simulink model "StateFlow_Control"  (R2025b)
settings: Solver=VariableStepAuto  StartTime=0.0  StopTime=514*8  RelTol=1e-3
libraries: slpidlib x1, simulink x1
settings Model: Creator=acer  LastModifiedBy=acer

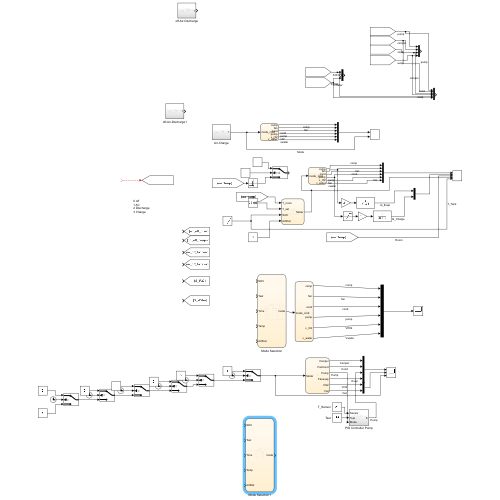
[thumbnail: Simulink's stored preview of the top-level diagram]
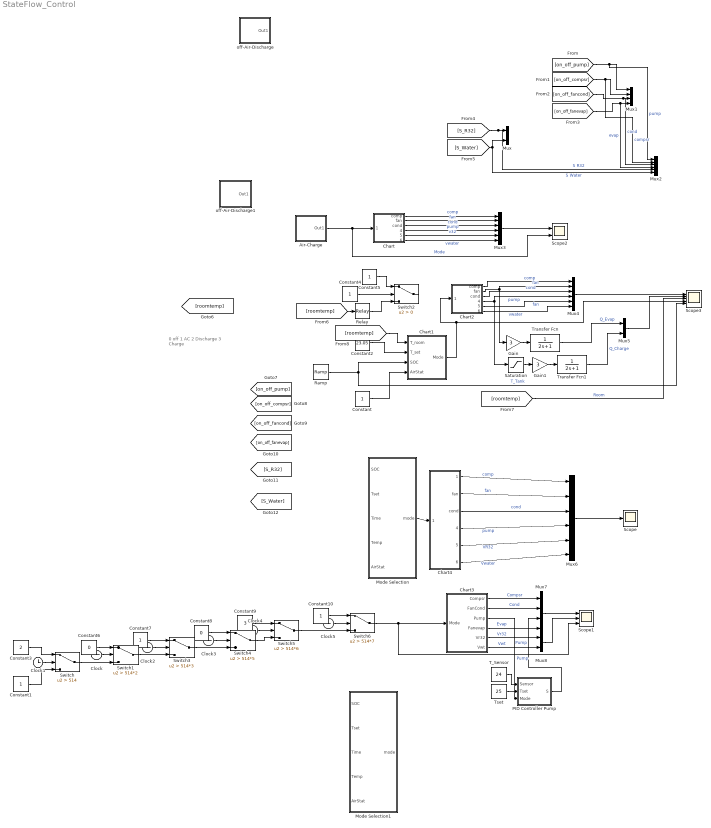
== system StateFlow_Control ==
  note: 0 off
      | 1 AC
      | 2 Discharge
      | 3 Charge
  Air-Charge : Subsystem
  Chart : Stateflow chart  TreatAsAtomicUnit=on
  Chart1 : Stateflow chart  TreatAsAtomicUnit=on
  Chart2 : Stateflow chart  TreatAsAtomicUnit=on
  Chart3 : Stateflow chart  TreatAsAtomicUnit=on
  Chart4 : Stateflow chart  TreatAsAtomicUnit=on
  Clock{,1..5} (6 alike) : Clock
  Constant{,1,4..5,7,10} (6 alike) : Constant
  Constant2 : Constant  Value=23.05
  Constant3 : Constant  Value=2
  Constant6 : Constant  Value=0
  Constant8 : Constant  Value=0
  Constant9 : Constant  Value=3
  Gain : Gain  Gain=3
  Gain1 : Gain  Gain=3
  Mode Selection : Stateflow chart  TreatAsAtomicUnit=on
  Mode Selection1 : Stateflow chart  TreatAsAtomicUnit=on
  Mux : Mux  Inputs=3
  Mux1 : Mux
  Mux{2..4,6} (4 alike) : Mux  Inputs=6
  Mux5 : Mux  Inputs=2
  Mux7 : Mux
  Mux8 : Mux  Inputs=2
  PID Controller Pump : Subsystem
  Ramp : simulink/Sources/Ramp  slope=-0.5/3600  start=950  InitialOutput=0.9
  Relay : Relay  OnSwitchValue=23.85  OffSwitchValue=23.05  OffOutputValue=3
  Saturation : Saturate  UpperLimit=100  LowerLimit=0
  Scope : Scope
      settings: ActiveDisplayYMinimum=-1  ActiveDisplayYMaximum=1
  Scope1 : Scope  NumInputPorts=3
      settings: ActiveDisplayYMinimum=-0.2604653153601002  ActiveDisplayYMaximum=0.35964334097048944
  Scope2 : Scope  NumInputPorts=2
      settings: ActiveDisplayYMinimum=-1  ActiveDisplayYMaximum=1  DataLoggingVariableName=ScopeData2
  Scope3 : Scope  NumInputPorts=5
      settings: ActiveDisplayYMinimum=-1.25  ActiveDisplayYMaximum=1.25  DataLoggingVariableName=ScopeData3
  Switch : Switch  Criteria=u2 > Threshold  Threshold=514  SaturateOnIntegerOverflow=off  InputSameDT=off
  Switch1 : Switch  Criteria=u2 > Threshold  Threshold=514*2  SaturateOnIntegerOverflow=off  InputSameDT=off
  Switch2 : Switch  Criteria=u2 > Threshold  SaturateOnIntegerOverflow=off  InputSameDT=off
  Switch3 : Switch  Criteria=u2 > Threshold  Threshold=514*3  SaturateOnIntegerOverflow=off  InputSameDT=off
  Switch4 : Switch  Criteria=u2 > Threshold  Threshold=514*5  SaturateOnIntegerOverflow=off  InputSameDT=off
  Switch5 : Switch  Criteria=u2 > Threshold  Threshold=514*6  SaturateOnIntegerOverflow=off  InputSameDT=off
  Switch6 : Switch  Criteria=u2 > Threshold  Threshold=514*7  SaturateOnIntegerOverflow=off  InputSameDT=off
  T_Sensor : Constant  Value=24
  Transfer Fcn : TransferFcn  Denominator=[2 1]
  Transfer Fcn1 : TransferFcn  Denominator=[2 1]
  Tset : Constant  Value=25
  off-Air-Discharge : Subsystem
  off-Air-Discharge1 : Subsystem
  wires:
  [S_R32] -> Mux2/5, Mux/1  "S R32"
  [S_Water] -> Mux2/6, Mux/3  "S Water"
  [on_off_fancond] -> Mux2/3, Mux1/3  "cond"
  [on_off_pump] -> Mux2/1, Mux1/1  "pump"
  [on_off_compsr] -> Mux2/2, Mux1/2  "compsr"
  [on_off_fanevap] -> Mux2/4, Mux1/4  "evap"
  Air-Charge/1(Out1) -> Scope2/2, Chart/1(mode_cmd)  "Mode"
  Chart/1(comp) -> Mux3/1  "comp"
  Chart/2(fan) -> Mux3/2  "fan"
  Chart/3(cond) -> Mux3/3  "cond"
  Chart/4(pump) -> Mux3/4  "pump"
  Chart/5(v_r32) -> Mux3/5  "v32"
  Chart/6(v_water) -> Mux3/6  "vwater"
  Mux3/1 -> Scope2/1
  Constant4/1 -> Switch2/2
  Constant5/1 -> Switch2/1
  Mux4/1 -> Scope3/1
  Chart2/3(cond) -> Mux4/3  "cond"
  Chart2/4(pump) -> Mux4/4, Saturation/1  "pump"
  Chart2/6(v_water) -> Mux4/6  "vwater"
  Chart2/1(comp) -> Mux4/1  "comp"
  Chart2/2(fan) -> Mux4/2, Gain/1  "fan"
  [roomtemp] -> Relay/1
  ? -> [roomtemp]
  Relay/1 -> Switch2/3
  Gain/1 -> Transfer Fcn/1
  Gain1/1 -> Transfer Fcn1/1
  Chart2/5(v_r32) -> Mux4/5  "fan"
  Transfer Fcn/1 -> Mux5/1  "Q_Evap"
  Transfer Fcn1/1 -> Mux5/2  "Q_Charge"
  Mux5/1 -> Scope3/2
  Saturation/1 -> Gain1/1
  [roomtemp] -> Scope3/3  "Room"
  [roomtemp] -> Chart1/1(T_room)
  Constant/1 -> Chart1/4(AirStat)
  Ramp/1 -> Chart1/3(SOC), Scope3/5  "T_Tank"
  Constant2/1 -> Chart1/2(T_set)
  Chart1/1(Mode) -> Scope3/4, Chart2/1(mode_cmd)
  Chart4/2(fan) -> Mux6/2  "fan"
  Chart4/4(pump) -> Mux6/4  "pump"
  Chart4/6(v_water) -> Mux6/6  "Vwater"
  Chart4/1(comp) -> Mux6/1  "comp"
  Mux6/1 -> Scope/1
  Chart4/5(v_r32) -> Mux6/5  "VR32"
  Chart4/3(cond) -> Mux6/3  "cond"
  Mode Selection/1(mode) -> Chart4/1(mode_cmd)
  Switch/1 -> Switch1/3
  Switch1/1 -> Switch3/3
  Clock/1 -> Switch1/2
  Clock1/1 -> Switch/2
  Clock2/1 -> Switch3/2
  Constant1/1 -> Switch/3
  Constant3/1 -> Switch/1
  Constant6/1 -> Switch1/1
  Constant7/1 -> Switch3/1
  Constant8/1 -> Switch4/1
  Switch3/1 -> Switch4/3
  Clock3/1 -> Switch4/2
  Switch4/1 -> Switch5/3
  Clock4/1 -> Switch5/2
  Constant9/1 -> Switch5/1
  Constant10/1 -> Switch6/1
  Clock5/1 -> Switch6/2
  Switch5/1 -> Switch6/3
  Chart3/1(Compsr) -> Mux7/1  "Compsr"
  Chart3/2(FanCond) -> Mux7/2  "Cond"
  Chart3/4(Fanevap) -> Mux7/4  "Evap"
  Chart3/5(Vr32) -> Mux8/1  "Vr32"
  Chart3/6(Vwt) -> Mux8/2  "Vwt"
  Mux7/1 -> Scope1/1
  Mux8/1 -> Scope1/2
  T_Sensor/1 -> PID Controller Pump/1(Sensor)
  Tset/1 -> PID Controller Pump/2(Tset)
  Switch6/1 -> Scope1/3, Chart3/1(Mode)
  Chart3/3(Pump) -> PID Controller Pump/3(Mode)  "Pump"
  PID Controller Pump/1(S) -> Mux7/3  "Pump"

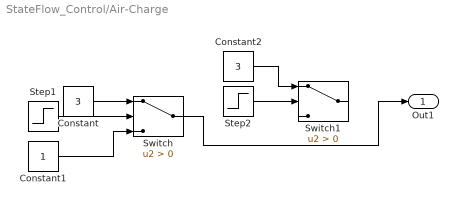
== system StateFlow_Control/Air-Charge ==
  Constant : Constant  Value=3
  Constant1 : Constant
  Constant2 : Constant  Value=3
  Step1 : Step  Time=15  SampleTime=0
  Step2 : Step  Time=20  SampleTime=0
  Switch : Switch  Criteria=u2 > Threshold  SaturateOnIntegerOverflow=off  InputSameDT=off
  Switch1 : Switch  Criteria=u2 > Threshold  SaturateOnIntegerOverflow=off  InputSameDT=off
  Out1 : Outport
  wires:
  Step1/1 -> Switch/2
  Step2/1 -> Switch1/2
  Constant/1 -> Switch/1
  Constant1/1 -> Switch/3
  Constant2/1 -> Switch1/1
  Switch/1 -> Out1/1

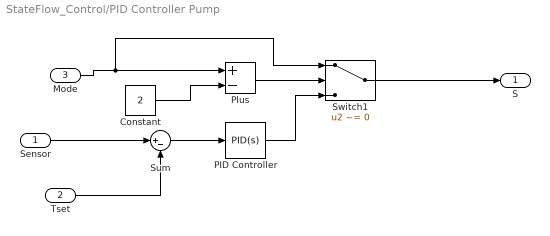
== system StateFlow_Control/PID Controller Pump ==
  Sensor : Inport
  Tset : Inport  Port=2
  Mode : Inport  Port=3
  Constant : Constant  Value=2
  PID Controller : slpidlib/PID Controller  Controller=PID  Form=Parallel  TimeDomain=Continuous-time  UseExternalTs=off  SampleTime=-1  IntegratorMethod=Forward Euler  FilterMethod=Forward Euler  ControllerParametersSource=internal  P=1  I=0.005  UseKiTs=off  D=0  UseExternalDerivativeSource=off  N=100  UseFilter=on  TunerSelectOption=Transfer Function Based (PID Tuner App)  InitialConditionSource=internal  InitialConditionForIntegrator=0  InitialConditionForFilter=0  DifferentiatorICPrevScaledInput=0  ExternalReset=none  TrackingMode=off  Kt=1  LimitOutput=off  SatLimitsSource=internal  UpperSaturationLimit=inf  LowerSaturationLimit=-inf  LinearizeAsGain=on  AntiWindupMode=none  Kb=1  LimitIntegrator=off  UpperIntegratorSaturationLimit=inf  LowerIntegratorSaturationLimit=-inf  POutMin=[]  POutMax=[]  IOutMin=[]  IOutMax=[]  DOutMin=[]  DOutMax=[]  NOutMin=[]  NOutMax=[]  SumOutMin=[]  SumOutMax=[]  SaturationOutMin=[]  SaturationOutMax=[]  PParamMin=[]  PParamMax=[]  IParamMin=[]  IParamMax=[]  DParamMin=[]  DParamMax=[]  NParamMin=[]  NParamMax=[]  KbParamMin=[]  KbParamMax=[]  KtParamMin=[]  KtParamMax=[]  KbOutMin=[]  KbOutMax=[]  KtOutMin=[]  KtOutMax=[]  IntegratorOutMin=[]  IntegratorOutMax=[]  FilterOutMin=[]  FilterOutMax=[]  SumI1OutMin=[]  SumI1OutMax=[]  SumI2OutMin=[]  SumI2OutMax=[]  SumI3OutMin=[]  SumI3OutMax=[]  SumI4OutMin=[]  SumI4OutMax=[]  SumDOutMin=[]  SumDOutMax=[]  DifferentiatorOutMin=[]  DifferentiatorOutMax=[]  FilterDiffOutCoefMin=[]  FilterDiffOutCoefMax=[]  ReciprocalOutMin=[]  ReciprocalOutMax=[]  SumDenOutMin=[]  SumDenOutMax=[]  SumNumOutMin=[]  SumNumOutMax=[]  DivideOutMin=[]  DivideOutMax=[]  UdiffTsProdOutMin=[]  UdiffTsProdOutMax=[]  NTsProdOutMin=[]  NTsProdOutMax=[]  UintegralTsProdOutMin=[]  UintegralTsProdOutMax=[]  UngainTsProdOutMin=[]  UngainTsProdOutMax=[]  ClampingZeroOutDataTypeStr=Inherit: Inherit via back propagation  ClampingZeroOutMin=[]  ClampingZeroOutMax=[]  FilterDenConstantOutDataTypeStr=Inherit: Inherit via back propagation  FilterDenConstantOutMin=[]  FilterDenConstantOutMax=[]  PCopyOutDataTypeStr=Inherit: Inherit via back propagation  PCopyOutMin=[]  PCopyOutMax=[]  NCopyOutDataTypeStr=Inherit: Inherit via back propagation  NCopyOutMin=[]  NCopyOutMax=[]  IntegratorContinuousStateAttributes=''  IntegratorStateMustResolveToSignalObject=off  IntegratorRTWStateStorageClass=Auto  FilterContinuousStateAttributes=''  FilterStateMustResolveToSignalObject=off  FilterRTWStateStorageClass=Auto  ParallelPVariant=InternalParameters  IdealPVariant=Disabled  IVariant=InternalParameters  DVariant=InternalParameters  IntegratorVariant=Continuous  SatVariant=Disabled  AWVariant=Passthrough  PCopyVariant=Disabled  TRVariant=Disabled  FdbkBlocksVariant=Forward  IdealPFdbkVariant=Disabled  SatFdbkVariant=Disabled  DerivativeFilterVariant=ContFilter  NVariant=InternalParameters  NCopyVariant=Disabled  FilterICVariant=InternalICsFilter  IntegratorICVariant=InternalICs  ExternalResetVariant=Disabled  TRSumVariant=Passthrough  SumFdbkVariant=Disabled  SumVariant=Sum_PID  TsampFilterVariant=InternalTs  TsampNgainVariant=Passthrough  TsampIntegralVariant=Disabled_SignalSpec  ExternalSaturationOutDataTypeStr=Inherit: Same as second input  DerivativeSourceVariant=ErrorSignal  PreIntVariant=InternalPreInt
  Plus : Sum  Inputs=+-
  Sum : Sum  Inputs=|+-
  Switch1 : Switch  Criteria=u2 ~= 0  Threshold=2  SaturateOnIntegerOverflow=off  InputSameDT=off
  S : Outport
  wires:
  Sensor/1 -> Sum/1
  Sum/1 -> PID Controller/1
  Switch1/1 -> S/1
  Tset/1 -> Sum/2
  Mode/1 -> Switch1/1, Plus/1
  Plus/1 -> Switch1/2
  Constant/1 -> Plus/2
  PID Controller/1 -> Switch1/3

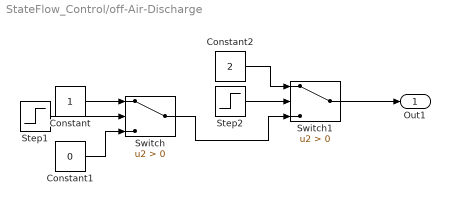
== system StateFlow_Control/off-Air-Discharge ==
  Constant : Constant
  Constant1 : Constant  Value=0
  Constant2 : Constant  Value=2
  Step1 : Step  Time=10  SampleTime=0
  Step2 : Step  Time=20  SampleTime=0
  Switch : Switch  Criteria=u2 > Threshold  SaturateOnIntegerOverflow=off  InputSameDT=off
  Switch1 : Switch  Criteria=u2 > Threshold  SaturateOnIntegerOverflow=off  InputSameDT=off
  Out1 : Outport
  wires:
  Step1/1 -> Switch/2
  Step2/1 -> Switch1/2
  Constant/1 -> Switch/1
  Switch1/1 -> Out1/1
  Constant1/1 -> Switch/3
  Switch/1 -> Switch1/3
  Constant2/1 -> Switch1/1

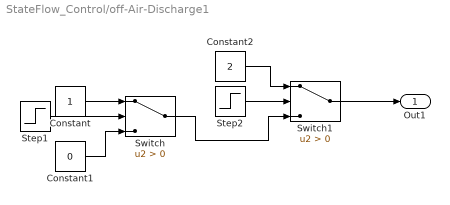
== system StateFlow_Control/off-Air-Discharge1 ==
  Constant : Constant
  Constant1 : Constant  Value=0
  Constant2 : Constant  Value=2
  Step1 : Step  Time=10  SampleTime=0
  Step2 : Step  Time=20  SampleTime=0
  Switch : Switch  Criteria=u2 > Threshold  SaturateOnIntegerOverflow=off  InputSameDT=off
  Switch1 : Switch  Criteria=u2 > Threshold  SaturateOnIntegerOverflow=off  InputSameDT=off
  Out1 : Outport
  wires:
  Step1/1 -> Switch/2
  Step2/1 -> Switch1/2
  Constant/1 -> Switch/1
  Switch1/1 -> Out1/1
  Constant1/1 -> Switch/3
  Switch/1 -> Switch1/3
  Constant2/1 -> Switch1/1

== stateflow chart StateFlow_Control/Chart ==
  state Mode_0
    entry: comp=0; fan=0; cond=0; pump=0; v_r32=1; v_water=-1;
  state Wait_Stat
    entry: comp=0; fan=0; cond=0; pump=0;
  state Mode_1_AC
    entry: comp=1; fan=1; cond=1; pump=0; v_r32=1; v_water=-1;
  state Mode_2_Discharge
    entry: comp=0; fan=1; cond=0; pump=1; v_r32=-1; v_water=1;
  state Mode_3_Charge
    entry: comp=1; fan=0; cond=1; pump=1; v_r32=-1; v_water=-1;
  (default) -> Mode_0
  Mode_0 -> Wait_Stat : [mode_cmd ~= 0]
  Wait_Stat -> Mode_0 [order 1] : [after(3, sec) && mode_cmd == 0]
  Mode_1_AC -> Wait_Stat : [mode_cmd ~= 1]
  Wait_Stat -> Mode_1_AC [order 2] : [after(3, sec) && mode_cmd == 1]
  Wait_Stat -> Mode_2_Discharge [order 3] : [after(3, sec) && mode_cmd == 2]
  Mode_2_Discharge -> Wait_Stat : [mode_cmd ~= 2 ]
  Mode_3_Charge -> Wait_Stat : [mode_cmd ~= 3 ]
  Wait_Stat -> Mode_3_Charge [order 4] : [after(3, sec) && mode_cmd == 3]
  data: mode_cmd input; comp output; fan output; cond output; pump output; v_r32 output; v_water output

== stateflow chart StateFlow_Control/Mode Selection ==
  state Charge_NoPeople
    entry : mode =2;ChargeStat = 1;
    during:
    if SOC >= 1
    ChargeStat = 1;
    else
    ChargeStat = 0;
    end
  state Main
    entry : mode = 0;warn = 0
  state Onpeak
    state On_Peak
      entry: mode = 0;
    state AC_Mode
      entry : mode = 1;
      if SOC > 0.5
      warn = 0;
      end
      during:
      if SOC > 0.5
      warn = 0;
      end
    state Discharge_Mode
      entry : mode = 2;
      exit: warn = 1
    AC_Mode -> On_Peak [order 2] : [warn == 1&& Temp <= Tset-0.5]
    On_Peak -> AC_Mode : [Temp>Tset-0.5]
    AC_Mode -> Discharge_Mode [order 1] : [Temp<Tset && SOC >0.5 && warn ==0]
    Discharge_Mode -> AC_Mode : [Temp>Tset+0.5 || SOC < 0.3]
  state Offpeak
    state Off_Peak
      entry: mode = 0;
      if SOC >= 1
      ChargeStat = 1;
      else
      ChargeStat = 0;
      end
    state AC_ModeNight
      entry: mode = 1;
      during:
      if SOC >= 1
      ChargeStat = 1;
      else
      ChargeStat = 0;
      end
    state Charge_Mode
      entry: mode = 3;
      during:
      if SOC >= 1
      ChargeStat = 1;
      end
    Off_Peak -> AC_ModeNight : [Temp>=Tset-0.5]
    AC_ModeNight -> Off_Peak [order 2] : [ChargeStat ==1&& Temp <= Tset-0.5]
    AC_ModeNight -> Charge_Mode [order 1] : [Temp <= Tset-0.5 && ChargeStat ==0]
    Charge_Mode -> AC_ModeNight : [Temp <= Tset-0.5 || ChargeStat ==1]
  (default) -> Main
  Main -> Charge_NoPeople [order 3] : [Time < 9 || Time>22 && AirStat ==2]
  Charge_NoPeople -> Main : [ChargeStat ==1|| AirStat ~=2]
  Onpeak -> Main : [AirStat == 0]
  Main -> On_Peak [order 1] : [9<Time<22&& AirStat==1]
  Offpeak -> Main : [AirStat == 0]
  Main -> Off_Peak [order 2] : [Time < 9 || Time>22 && AirStat ==1]
  data: SOC input; Tset input; Time input; Temp input; AirStat input; warn local; ChargeStat local; mode output

== stateflow chart StateFlow_Control/Chart4 ==
  state Mode_0
    entry: comp=0; fan=0; cond=0; pump=0; v_r32=1; v_water=-1;
  state Wait_Stat
    entry: comp=0; fan=0; cond=0; pump=0;
  state Mode_1_AC
    entry: comp=1; fan=1; cond=1; pump=0; v_r32=1; v_water=-1;
  state Mode_2_Discharge
    entry: comp=0; fan=1; cond=0; pump=1; v_r32=-1; v_water=1;
  state Mode_3_Charge
    entry: comp=1; fan=0; cond=1; pump=1; v_r32=-1; v_water=-1;
  (default) -> Mode_0
  Mode_0 -> Wait_Stat : [mode_cmd ~= 0]
  Wait_Stat -> Mode_0 [order 1] : [after(3, sec) && mode_cmd == 0]
  Mode_1_AC -> Wait_Stat : [mode_cmd ~= 1]
  Wait_Stat -> Mode_1_AC [order 2] : [after(3, sec) && mode_cmd == 1]
  Wait_Stat -> Mode_2_Discharge [order 3] : [after(3, sec) && mode_cmd == 2]
  Mode_2_Discharge -> Wait_Stat : [mode_cmd ~= 2 ]
  Mode_3_Charge -> Wait_Stat : [mode_cmd ~= 3 ]
  Wait_Stat -> Mode_3_Charge [order 4] : [after(3, sec) && mode_cmd == 3]
  data: mode_cmd input; comp output; fan output; cond output; pump output; v_r32 output; v_water output

== stateflow chart StateFlow_Control/Chart3 ==
  state Mode0
    entry : Compsr = 0; Fanevap =0;
    FanCond = 0 ;Pump = 0;Vr32 =1; Vwt=-1;P=0
  state Wait_State
    entry : Compsr = 0; Fanevap =0;
    FanCond = 0;Pump=0 ; P=1
  state Valve_Control_3
    entry : Vr32 =-1; Vwt=1;P=0
  state Mode3_Charge
    entry : Compsr = 1; Fanevap =0;
    FanCond = 1 ;Pump = 1;P=0
  state Mode1_AC
    entry : Compsr = 0.9; Fanevap =0.8;
    FanCond = 0.9 ;Pump=0;P=0
  state Valve_Control_1
    entry : Vr32 =1; Vwt=-1;P=0
  state Valve_Control_2
    entry : Vr32 =-1; Vwt=1;P=0
  state Mode2_Discharge
    entry : Compsr = 0; Fanevap =0.3;
    FanCond = 0 ;Pump = 2;P=0
  (default) -> Mode0
  Wait_State -> Mode0 [order 1] : [Mode ==0]
  Mode0 -> Wait_State : [Mode~=0]
  Wait_State -> Valve_Control_3 [order 4] : [after(1,sec) && Mode ==3]
  Mode1_AC -> Wait_State : [Mode~=1]
  Valve_Control_3 -> Mode3_Charge : [P==0&&after(0.5,sec) ]
  Mode3_Charge -> Wait_State : [Mode~=3]
  Wait_State -> Valve_Control_1 [order 3] : [after(1,sec) &&P==1&& Mode ==1]
  Valve_Control_1 -> Mode1_AC : [P==0&&after(0.5,sec) ]
  Mode2_Discharge -> Wait_State : [Mode~=2]
  Wait_State -> Valve_Control_2 [order 2] : [after(1,sec) &&P==1&& Mode ==2]
  Valve_Control_2 -> Mode2_Discharge : [P==0&&after(0.5,sec) ]
  data: Mode input; Compsr output; FanCond output; Pump output; Fanevap output; Vr32 output; P local; Vwt output

== stateflow chart StateFlow_Control/Mode Selection1 ==
  state ChangeValve
    entry : Vr32=-1;Vwater=-1
  state Charge_NoPeople
    entry : mode =2;ChargeStat = 1;
    Compsr=2;
    Cond=2;Evap=0;Pump=1;
    during:
    if SOC >= 1
    ChargeStat = 1;
    else
    ChargeStat = 0;
    end
  state Main
    entry : mode = 0;warn = 0;Compsr=0;
    Cond=0;Evap=0;Pump=0;
  state Onpeak
    state On_Peak
      entry: mode = 0;
    state AC_Mode
      entry : mode = 1;Compsr=1;Cond=1;Evap=0.8;Pump=0;
      if SOC > 0.5
      warn = 0;
      end
      during:
      if SOC > 0.5
      warn = 0;
      end
    state Discharge_Mode
      entry : mode = 2;
      exit: warn = 1
    AC_Mode -> On_Peak [order 2] : [warn == 1&& Temp <= Tset-0.5]
    On_Peak -> AC_Mode : [Temp>Tset-0.5]
    AC_Mode -> Discharge_Mode [order 1] : [Temp<Tset && SOC >0.5 && warn ==0]
    Discharge_Mode -> AC_Mode : [Temp>Tset+0.5 || SOC < 0.3]
  state Offpeak
    state Off_Peak
      entry: mode = 0;
      if SOC >= 1
      ChargeStat = 1;
      else
      ChargeStat = 0;
      end
    state AC_ModeNight
      entry: mode = 1;
      during:
      if SOC >= 1
      ChargeStat = 1;
      else
      ChargeStat = 0;
      end
    state Charge_Mode
      entry: mode = 3;
      during:
      if SOC >= 1
      ChargeStat = 1;
      end
    Off_Peak -> AC_ModeNight : [Temp>=Tset-0.5]
    AC_ModeNight -> Off_Peak [order 2] : [ChargeStat ==1&& Temp <= Tset-0.5]
    AC_ModeNight -> Charge_Mode [order 1] : [Temp <= Tset-0.5 && ChargeStat ==0]
    Charge_Mode -> AC_ModeNight : [Temp <= Tset-0.5 || ChargeStat ==1]
  (default) -> Main
  ChangeValve -> Charge_NoPeople
  Main -> ChangeValve [order 3] : [Time < 9 || Time>22 && AirStat ==2]
  Charge_NoPeople -> Main : [ChargeStat ==1|| AirStat ~=2]
  Onpeak -> Main : [AirStat == 0]
  Main -> On_Peak [order 1] : [9<Time<22&& AirStat==1]
  Offpeak -> Main : [AirStat == 0]
  Main -> Off_Peak [order 2] : [Time < 9 || Time>22 && AirStat ==1]
  data: SOC input; Tset input; Time input; Temp input; AirStat input; warn local; ChargeStat local; mode output

== stateflow chart StateFlow_Control/Chart1 ==
  state Off
    entry : Mode =0;
  state Discharge
    entry : Mode=2;
  state AC
    entry : Mode = 1 ;
  (default) -> Off
  Off -> AC : [AirStat == 1 && T_room > T_set]
  AC -> Off [order 2] : [AirStat == 0]
  Discharge -> Off [order 2] : [AirStat == 0]
  AC -> Discharge [order 1] : [(SOC>0.3 && T_set == T_room) && AirStat == 1]
  Discharge -> AC [order 1] : [SOC <=0.3 || T_room >( T_set+1) && AirStat == 1]
  data: T_room input; T_set input; SOC input; Mode output; AirStat input

== stateflow chart StateFlow_Control/Chart2 ==
  state Mode_0
    entry: comp=0; fan=0; cond=0; pump=0; v_r32=1; v_water=-1;
  state Wait_Stat
    entry: comp=0; fan=0; cond=0; pump=0;
  state Mode_1_AC
    entry: comp=1; fan=1; cond=1; pump=0; v_r32=1; v_water=-1;
  state Mode_2_Discharge
    entry: comp=0; fan=1; cond=0; pump=1; v_r32=-1; v_water=1;
  state Mode_3_Charge
    entry: comp=1; fan=0; cond=1; pump=1; v_r32=-1; v_water=-1;
  (default) -> Mode_0
  Mode_0 -> Wait_Stat : [mode_cmd ~= 0]
  Wait_Stat -> Mode_0 [order 1] : [after(3, sec) && mode_cmd == 0]
  Mode_1_AC -> Wait_Stat : [mode_cmd ~= 1]
  Wait_Stat -> Mode_1_AC [order 2] : [after(3, sec) && mode_cmd == 1]
  Wait_Stat -> Mode_2_Discharge [order 3] : [after(3, sec) && mode_cmd == 2]
  Mode_2_Discharge -> Wait_Stat : [mode_cmd ~= 2 ]
  Mode_3_Charge -> Wait_Stat : [mode_cmd ~= 3 ]
  Wait_Stat -> Mode_3_Charge [order 4] : [after(3, sec) && mode_cmd == 3]
  data: mode_cmd input; comp output; fan output; cond output; pump output; v_r32 output; v_water output
